simulink model "Triggered_Subsystem"  (R2017b)
settings: Solver=FixedStepDiscrete  StartTime=0.0  StopTime=10.0  FixedStep=0.200000  RelTol=1e-3
settings Model: Creator=hbourbou  LastModifiedBy=hbourbou
settings DataIOCC: SaveFormat=StructureWithTime
settings OptimizationCC: LifeSpan=inf
settings DebuggingCC: SFExecutionAtInitializationDiag=none
settings HardwareCC: ProdBitPerSizeT=32  ProdBitPerPtrDiffT=32  ProdWordSize=32  ProdHWDeviceType=Specified
settings CodeAppCC: StateflowObjectComments=on

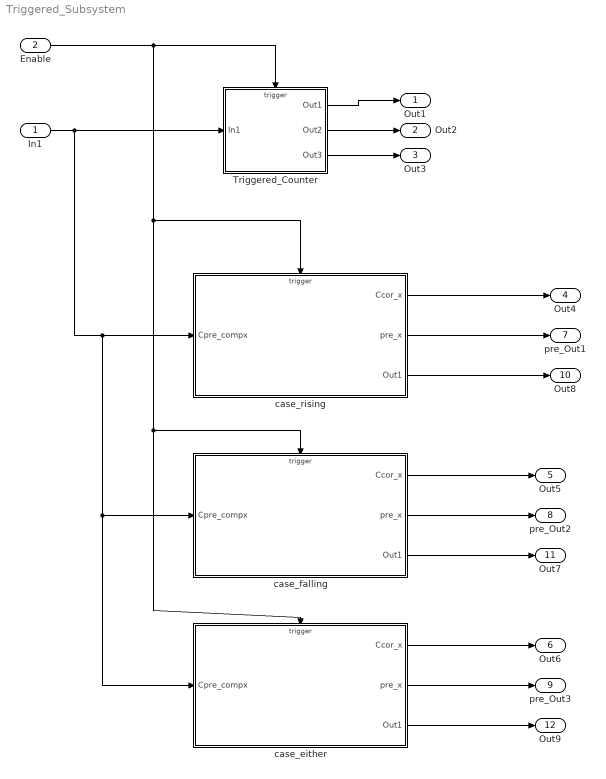
== system Triggered_Subsystem ==
  In1 : Inport
  Enable : Inport  Port=2
  Triggered_Counter : Subsystem  TreatAsAtomicUnit=on
  case_either : Subsystem  TreatAsAtomicUnit=on
  case_falling : Subsystem  TreatAsAtomicUnit=on
  case_rising : Subsystem  TreatAsAtomicUnit=on
  Out1 : Outport
  Out2 : Outport  Port=2
  Out3 : Outport  Port=3
  Out4 : Outport  Port=4
  Out5 : Outport  Port=5
  Out6 : Outport  Port=6
  pre_Out1 : Outport  Port=7
  pre_Out2 : Outport  Port=8
  pre_Out3 : Outport  Port=9
  Out8 : Outport  Port=10
  Out7 : Outport  Port=11
  Out9 : Outport  Port=12
  wires:
  Triggered_Counter/1(Out1) -> Out1/1
  Triggered_Counter/2(Out2) -> Out2/1
  Triggered_Counter/3(Out3) -> Out3/1
  Enable/1 -> Triggered_Counter/Trigger, case_rising/Trigger, case_falling/Trigger, case_either/Trigger
  case_rising/1(Ccor_x) -> Out4/1
  In1/1 -> Triggered_Counter/1(In1), case_either/1(Cpre_compx), case_falling/1(Cpre_compx), case_rising/1(Cpre_compx)
  case_falling/1(Ccor_x) -> Out5/1
  case_either/1(Ccor_x) -> Out6/1
  case_rising/2(pre_x) -> pre_Out1/1
  case_falling/2(pre_x) -> pre_Out2/1
  case_either/2(pre_x) -> pre_Out3/1
  case_rising/3(Out1) -> Out8/1
  case_falling/3(Out1) -> Out7/1
  case_either/3(Out1) -> Out9/1

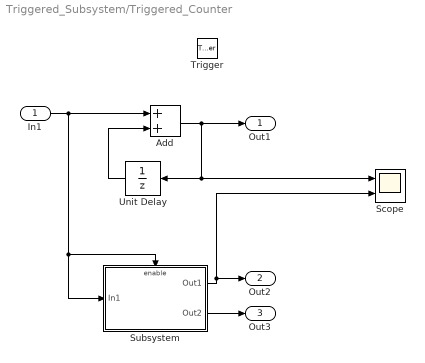
== system Triggered_Subsystem/Triggered_Counter ==
  In1 : Inport
  Trigger : TriggerPort  VariantControl=(inherit)  PortDimensions=1
  Add : Sum
  Scope : Scope  NumInputPorts=2
  Subsystem : Subsystem  TreatAsAtomicUnit=on
  Unit Delay : UnitDelay  SampleTime=-1
  Out1 : Outport  OutputWhenDisabled=reset  InitialOutput=0
  Out2 : Outport  Port=2
  Out3 : Outport  Port=3
  wires:
  Unit Delay/1 -> Add/2
  Subsystem/1(Out1) -> Scope/2, Out2/1
  In1/1 -> Subsystem/Enable, Subsystem/1(In1), Add/1
  Add/1 -> Scope/1, Unit Delay/1, Out1/1
  Subsystem/2(Out2) -> Out3/1

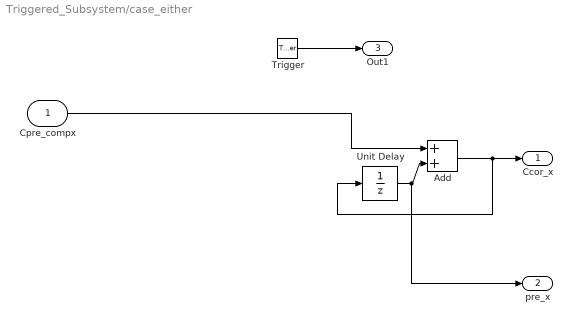
== system Triggered_Subsystem/case_either ==
  Cpre_compx : Inport  OutDataTypeStr=double  PortDimensions=[1]
  Trigger : TriggerPort  TriggerType=either  VariantControl=(inherit)  ShowOutputPort=on  PortDimensions=1
  Add : Sum
  Unit Delay : UnitDelay  SampleTime=-1.0000000000000000
  Ccor_x : Outport  InitialOutput=0
  pre_x : Outport  Port=2  InitialOutput=0
  Out1 : Outport  Port=3
  wires:
  Cpre_compx/1 -> Add/1
  Add/1 -> Unit Delay/1, Ccor_x/1
  Unit Delay/1 -> pre_x/1, Add/2
  Trigger/1 -> Out1/1

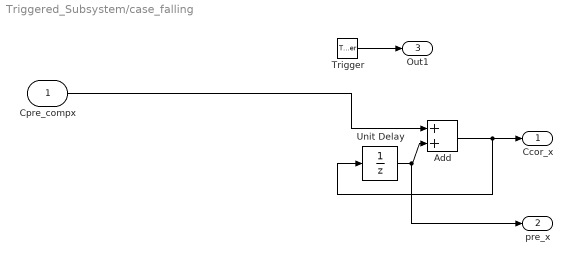
== system Triggered_Subsystem/case_falling ==
  Cpre_compx : Inport  OutDataTypeStr=double  PortDimensions=[1]
  Trigger : TriggerPort  TriggerType=falling  VariantControl=(inherit)  ShowOutputPort=on  PortDimensions=1
  Add : Sum
  Unit Delay : UnitDelay  SampleTime=-1.0000000000000000
  Ccor_x : Outport  OutputWhenDisabled=reset  InitialOutput=0
  pre_x : Outport  Port=2  InitialOutput=0
  Out1 : Outport  Port=3
  wires:
  Cpre_compx/1 -> Add/1
  Add/1 -> Unit Delay/1, Ccor_x/1
  Unit Delay/1 -> pre_x/1, Add/2
  Trigger/1 -> Out1/1

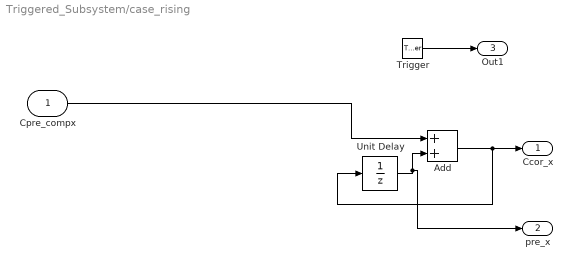
== system Triggered_Subsystem/case_rising ==
  Cpre_compx : Inport  OutDataTypeStr=double  PortDimensions=[1]
  Trigger : TriggerPort  VariantControl=(inherit)  ShowOutputPort=on  PortDimensions=1
  Add : Sum
  Unit Delay : UnitDelay  SampleTime=-1.0000000000000000
  Ccor_x : Outport  InitialOutput=0
  pre_x : Outport  Port=2  InitialOutput=0
  Out1 : Outport  Port=3
  wires:
  Cpre_compx/1 -> Add/1
  Unit Delay/1 -> pre_x/1, Add/2
  Add/1 -> Unit Delay/1, Ccor_x/1
  Trigger/1 -> Out1/1

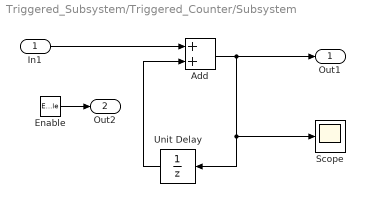
== system Triggered_Subsystem/Triggered_Counter/Subsystem ==
  In1 : Inport
  Enable : EnablePort  StatesWhenEnabling=reset  ShowOutputPort=on
  Add : Sum
  Scope : Scope
  Unit Delay : UnitDelay  SampleTime=-1
  Out1 : Outport
  Out2 : Outport  Port=2
  wires:
  In1/1 -> Add/1
  Unit Delay/1 -> Add/2
  Add/1 -> Scope/1, Unit Delay/1, Out1/1
  Enable/1 -> Out2/1
